simulink model "playback_mech_explorer"  (R2023b)
settings: Solver=VariableStepAuto  StartTime=0.0  StopTime=1  RelTol=1e-3
model workspace (MAT data in the model file):
  obstacle_enable = Simulink.Parameter
  obstacle_enable.Value = 0
  obstacle_enable.DataType = 'boolean'
  obstacle_enable.DocUnits = '1'
  obstacle_enable.Complexity = 'real'
  obstacle_enable.Dimensions = [1 1]
  pendulum_type = Simulink.Parameter
  pendulum_type.Value = 1
  pendulum_type.DataType = 'uint8'
  pendulum_type.DocUnits = '1'
  pendulum_type.Complexity = 'real'
  pendulum_type.Dimensions = [1 1]
undefined symbols (not defined in the file): pendulum_mass, Ts
libraries: fl_lib x2
settings Model: DataDictionary=data_interface.sldd  Creator=upattacini  LastModifiedBy=upattacini
settings DataIOCC: SaveOutput=off  SignalLogging=off  DSMLogging=off  SaveTime=off  ReturnWorkspaceOutputs=off
settings ExplorerConfigSet: InternalSimMechanicsExplorerSettings="<ExplorerConfiguration><canonicalview>default</canonicalview><AnimationSetting><BasePlaybackSpeed>1.0</BasePlaybackSpeed><PlaybackSpeedFactor>1.0</PlaybackSpeedFactor></AnimationSetting><TilePanel><TileInfo><Tiles Columns=\"1\" Count=\"1\" Rows=\"1\"><Column Weight=\"1\"/><Row Weight=\"1\"/><Tile Height=\"1\" Width=\"1\" X=\"0\" Y=\"0\"/></Tiles></TileInfo><SceneInfo><SceneViewer><BGColor><R>0.60000002384185791</R><G>0.60000002384185791</G><B>0.60000002384185791</B></BGColor><Camera><DoPerspective>off</DoPerspective><Position><X>0.0138410343925078685</X><Y>-0.282265129449846885</Y><Z>1.00000000000000022</Z></Position><Center><X>0.0138410343925078685</X><Y>-0.282265129449846885</Y><Z>2.22044604925031308e-16</Z></Center><Up><X>0</X><Y>1</Y><Z>-0</Z></Up><ViewLimDist>1</ViewLimDist><YLim>0.631458368488044708</YLim><XLim>0.844014048337693001</XLim></Camera></SceneViewer></SceneInfo></TilePanel><MechEditorPanel><Cameras/><GfxPanelCameraMap/><VideoCreator><PlaybackSpeedRatio>1.0</PlaybackSpeedRatio><FrameRate>30</FrameRate><VideoFormat>Motion JPEG AVI</VideoFormat><FrameSize>auto</FrameSize></VideoCreator></MechEditorPanel></ExplorerConfiguration>"

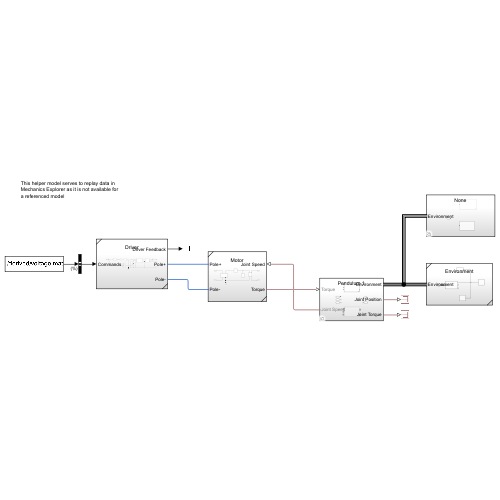
[thumbnail: Simulink's stored preview of the top-level diagram]
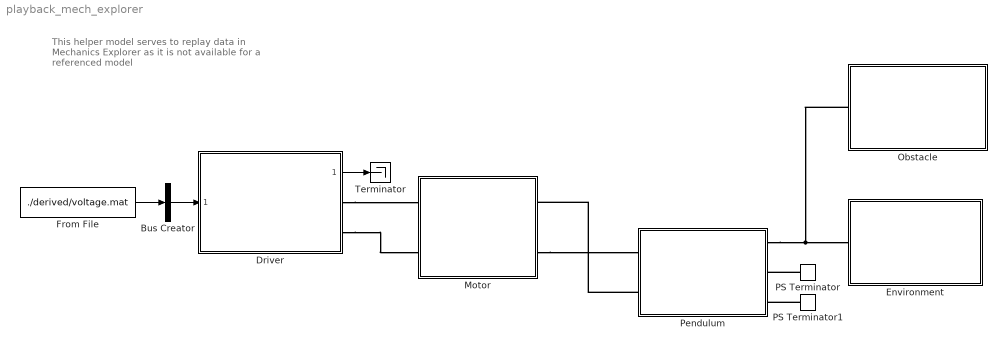
== system playback_mech_explorer ==
  note: This helper model serves to replay data in
      | Mechanics Explorer as it is not available for
      | a referenced model
  Bus Creator : BusCreator  Inputs=1  OutDataTypeStr=Bus: Control_Command  NonVirtualBus=on
      settings: InheritFromInputs=off
  Driver : Subsystem  ReferencedSubsystem=Driver
      settings: PermitHierarchicalResolution=None
  Environment : Subsystem  ReferencedSubsystem=Environment
      settings: PermitHierarchicalResolution=None
  From File : FromFile  FileName=./derived/voltage.mat  SampleTime=Ts  ExtrapolationBeforeFirstDataPoint=Hold first value  InterpolationWithinTimeRange=Zero order hold  ExtrapolationAfterLastDataPoint=Hold last value
  Motor : Subsystem  ReferencedSubsystem=Motor
      settings: PermitHierarchicalResolution=None
  Obstacle : Subsystem  Variant=on  VariantControl=Obstacle
  PS Terminator : fl_lib/Physical Signals/Sinks/PS Terminator
  PS Terminator1 : fl_lib/Physical Signals/Sinks/PS Terminator
  Pendulum : Subsystem  Variant=on  VariantControl=Pendulum
  Terminator : Terminator
  wires:
  From File/1 -> Bus Creator/1
  Bus Creator/1 -> Driver/1
  Driver/1 -> Terminator/1
  connections:
  Pendulum/LConn1 -- Obstacle/LConn1 -- Environment/LConn1
  PS Terminator/LConn1 -- Pendulum/LConn2
  PS Terminator1/LConn1 -- Pendulum/LConn3
  Pendulum/RConn2 -- Motor/RConn1
  Motor/RConn2 -- Pendulum/RConn1
  Driver/RConn1 -- Motor/LConn1
  Driver/RConn2 -- Motor/LConn2

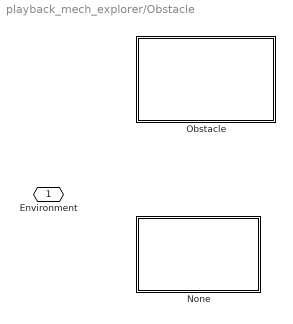
== system playback_mech_explorer/Obstacle ==
  None : Subsystem  VariantControl=obstacle_enable == false
  Obstacle : Subsystem  VariantControl=obstacle_enable == true  ReferencedSubsystem=Obstacle  l=0.5  m=0.1
      settings: PermitHierarchicalResolution=None
  Environment : PMIOPort  Side=Left

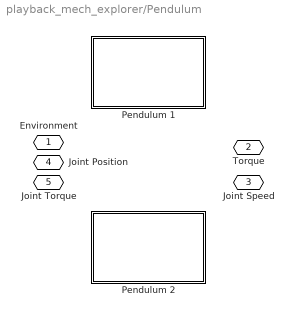
== system playback_mech_explorer/Pendulum ==
  Pendulum 1 : Subsystem  VariantControl=pendulum_type == 1  ReferencedSubsystem=Pendulum  l=pendulum_1_length  m=pendulum_mass
      settings: PermitHierarchicalResolution=None
  Pendulum 2 : Subsystem  VariantControl=pendulum_type == 2  ReferencedSubsystem=Pendulum  l=pendulum_2_length  m=pendulum_mass
      settings: PermitHierarchicalResolution=None
  Environment : PMIOPort  Side=Left
  Torque : PMIOPort  Port=2  Side=Right
  Joint Speed : PMIOPort  Port=3  Side=Right
  Joint Position : PMIOPort  Port=4  Side=Left
  Joint Torque : PMIOPort  Port=5  Side=Left

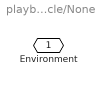
== system playback_mech_explorer/Obstacle/None ==
  Environment : PMIOPort  Side=Left
